simulink model "SquatTrotClimbRefined"  (R2025b)
settings: Solver=ode45  StartTime=0.0  StopTime=200  MaxStep=0.002  RelTol=0.01  AbsTol=0.01  EnableMultiTasking=on
undefined symbols (not defined in the file): a, b, c, waypoints, X, Y, Z
libraries: sm_lib x81, nesl_utility x67, hdlsllib x12, slpidlib x2, robotalgslib x1, sharedtransform x1
(part 4 of 6)

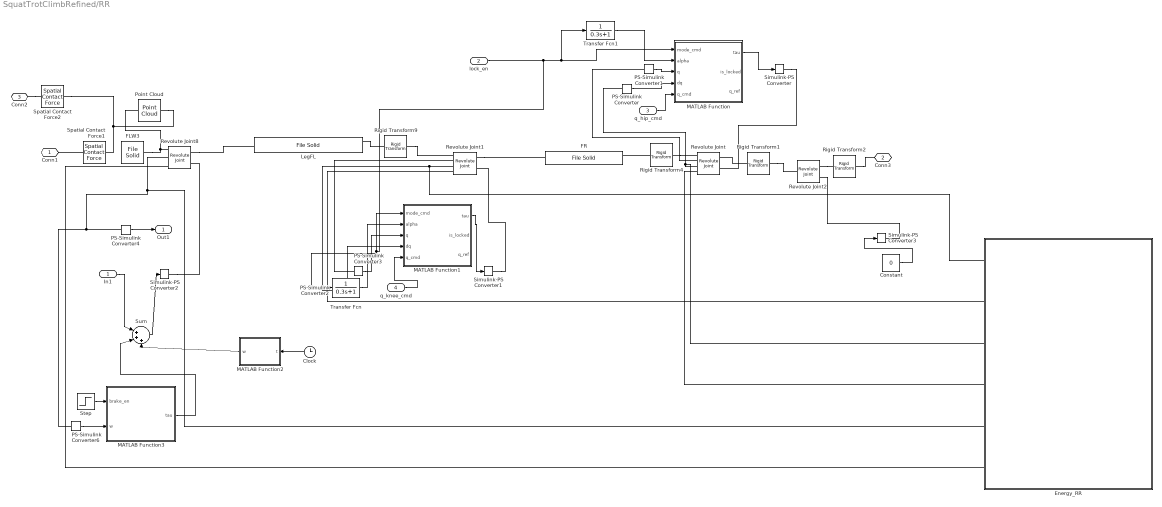
== system SquatTrotClimbRefined/RR ==
  In1 : Inport
  lock_en : Inport  Port=2
  q_hip_cmd : Inport  Port=3
  q_knee_cmd : Inport  Port=4
  Clock : Clock
  Constant : Constant  Value=0
  Energy_RR : Subsystem
  FLW3 : sm_lib/Body Elements/File Solid  ExtGeomFileName=Cheng Shin C-166-1.stp  UnitType=FromFile  ExtGeomFileUnits=m  StepReaderType=HEX  ExportConvexHullGeometry=on  InertiaType=CalculateFromGeometry  BasedOnType=Density  Density=400  DensityUnits=kg/m^3  Mass=1  MassUnits=kg  CenterOfMass=[0 0 0]  CenterOfMassUnits=m  MomentsOfInertia=[1 1 1]  MomentsOfInertiaUnits=kg*m^2  ProductsOfInertia=[0 0 0]  ProductsOfInertiaUnits=kg*m^2  GraphicType=FromGeometry  MarkerShape=Sphere  MarkerSize=10  GraphicVisPropType=AdvancedVisualProperties  GraphicDiffuseColor=[0.1 0.1 0.1]  GraphicOpacity=1  GraphicSpecularColor=[0.2 0.2 0.2 1.0]  GraphicAmbientColor=[0.05 0.05 0.05 1.0]  GraphicEmissiveColor=[0.0 0.0 0.0 1.0]  GraphicShininess=10  DoExposeReferenceFrame=off  SerializedFrames=<Frames><Frame><Id>Frame1</Id><Value><Name>F1</Name><Origin><Source>CenterOfMassFrame</Source><FeatureName>toroidal surface 99</FeatureName></Origin><PrimaryAxis><DefinedDirection>+Z</DefinedDirection><Source>ReferenceFrame</Source><SourceDirection>+Z</SourceDirection><FeatureName></FeatureName></PrimaryAxis><SecondaryAxis><DefinedDirection>+X</DefinedDirection><Source>ReferenceFrame</Source><SourceDirection>+X</SourceDirection><FeatureName></FeatureName></SecondaryAxis></Value></Frame></Frames>
  FR : sm_lib/Body Elements/File Solid  ExtGeomFileName=haut patte D.STEP  UnitType=FromFile  ExtGeomFileUnits=m  StepReaderType=HEX  ExportConvexHullGeometry=on  InertiaType=CalculateFromGeometry  BasedOnType=Density  Density=800  DensityUnits=kg/m^3  Mass=1  MassUnits=kg  CenterOfMass=[0 0 0]  CenterOfMassUnits=m  MomentsOfInertia=[1 1 1]  MomentsOfInertiaUnits=kg*m^2  ProductsOfInertia=[0 0 0]  ProductsOfInertiaUnits=kg*m^2  GraphicType=FromGeometry  MarkerShape=Sphere  MarkerSize=10  GraphicVisPropType=AdvancedVisualProperties  GraphicDiffuseColor=[0.9 0.9 0.9]  GraphicOpacity=1  GraphicSpecularColor=[0.9 0.9 0.9 1.0]  GraphicAmbientColor=[0.1 0.1 0.1 1.0]  GraphicEmissiveColor=[0.0 0.0 0.0 1.0]  GraphicShininess=100  DoExposeReferenceFrame=off  SerializedFrames=<Frames><Frame><Id>Frame1</Id><Value><Name>H-L link</Name><Origin><Source>GeometricFeature</Source><FeatureName>spherical surface 2</FeatureName></Origin><PrimaryAxis><DefinedDirection>+Z</DefinedDirection><Source>ReferenceFrame</Source><SourceDirection>+Z</SourceDirection><FeatureName></FeatureName></PrimaryAxis><SecondaryAxis><DefinedDirection>+X</DefinedDirection><Source>ReferenceFrame</Source><SourceDirection>-Y</SourceDirection><FeatureName></FeatureName></SecondaryAxis></Value></Frame><Frame><Id>Frame2</Id><Value><Name>L-K link</Name><Origin><Source>GeometricFeature</Source><FeatureName>cylindrical surface 2</FeatureName></Origin><PrimaryAxis><DefinedDirection>+Z</DefinedDirection><Source>ReferenceFrame</Source><SourceDirection>+Z</SourceDirection><FeatureName></FeatureName></PrimaryAxis><SecondaryAxis><DefinedDirection>+X</DefinedDirection><Source>ReferenceFrame</Source><SourceDirection>-Y</SourceDirection><FeatureName></FeatureName></SecondaryAxis></Value></Frame></Frames>
  LegFL : sm_lib/Body Elements/File Solid  ExtGeomFileName=leg.STEP  UnitType=FromFile  ExtGeomFileUnits=m  StepReaderType=HEX  ExportConvexHullGeometry=on  InertiaType=CalculateFromGeometry  BasedOnType=Density  Density=800  DensityUnits=kg/m^3  Mass=1  MassUnits=kg  CenterOfMass=[0 0 0]  CenterOfMassUnits=m  MomentsOfInertia=[1 1 1]  MomentsOfInertiaUnits=kg*m^2  ProductsOfInertia=[0 0 0]  ProductsOfInertiaUnits=kg*m^2  GraphicType=FromGeometry  MarkerShape=Sphere  MarkerSize=10  GraphicVisPropType=AdvancedVisualProperties  GraphicDiffuseColor=[0 0 0]  GraphicOpacity=1  GraphicSpecularColor=[0.9 0.9 0.9 1.0]  GraphicAmbientColor=[0.1 0.1 0.1 1.0]  GraphicEmissiveColor=[0.0 0.0 0.0 1.0]  GraphicShininess=100  DoExposeReferenceFrame=off  SerializedFrames=|
      | <Frames>
      | 
      |   <Frame>
      |     <Id>Frame1</Id>
      |     <Value>
      |       <Name>L-K link</Name>
      |       <Origin>
      |         <Source>GeometricFeature</Source>
      |         <FeatureName>cylindrical surface 6</FeatureName>
      |       </Origin>
      |       <PrimaryAxis>
      |         <DefinedDirection>+Z</DefinedDirection>
      |         <Source>ReferenceFrame</Source>
      |         <SourceDirection>+Z</SourceDirection>
      |         <FeatureName></FeatureName>
      |       </PrimaryAxis>
      |       <SecondaryAxis>
      |         <DefinedDirection>+X</DefinedDirection>
      |         <Source>ReferenceFrame</Source>
      |         <SourceDirection>-X</SourceDirection>
      |         <FeatureName></FeatureName>
      |       </SecondaryAxis>
      |     </Value>
      |   </Frame>
      | 
      |   <Frame>
      |     <Id>Frame2</Id>
      |     <Value>
      |       <Name>L-W link</Name>
      |       <Origin>
      |         <Source>GeometricFeature</Source>
      |         <FeatureName>cylindrical surface 4</FeatureName>
      |       </Origin>
      |       <PrimaryAxis>
      |         <DefinedDirection>+Z</DefinedDirection>
      |         <Source>ReferenceFrame</Source>
      |         <SourceDirection>+Z</SourceDirection>
      |         <FeatureName></FeatureName>
      |       </PrimaryAxis>
      |       <SecondaryAxis>
      |         <DefinedDirection>+X</DefinedDirection>
      |         <Source>ReferenceFrame</Source>
      |         <SourceDirection>-X</SourceDirection>
      |         <FeatureName></FeatureName>
      |       </SecondaryAxis>
      |     </Value>
      |   </Frame>
      | 
      | </Frames>
  MATLAB Function : MATLAB Function  TreatAsAtomicUnit=on  SystemSampleTime=0.002
  MATLAB Function1 : MATLAB Function  TreatAsAtomicUnit=on  SystemSampleTime=0.002
  MATLAB Function2 : MATLAB Function  TreatAsAtomicUnit=on
  MATLAB Function3 : MATLAB Function  TreatAsAtomicUnit=on
  PS-Simulink Converter{,1..4,6} (6 alike) : nesl_utility/PS-Simulink Converter  PhysicalDomain=network_engine_domain  SubClassName=ps_output  LeftPortType=input  RightPortType=output  PseudoPeriodic=off  Frequencies=[]  VectorFormat=inherit  Unit=inherit  AffineConversion=off
  Point Cloud : sm_lib/Curves and Surfaces/Point Cloud  CoordinatesMatrix=wheel_pts  CoordinatesMatrixUnits=m  GraphicType=MarkerCloud  GraphicSphereRadius=1e-2  GraphicSphereRadiusUnits=m  GraphicVisPropType=SimpleVisualProperties  GraphicDiffuseColor=[0.5 0.5 0.5]  GraphicOpacity=1  GraphicSpecularColor=[0.5 0.5 0.5 1.0]  GraphicAmbientColor=[0.15 0.15 0.15 1.0]  GraphicEmissiveColor=[0.0 0.0 0.0 1.0]  GraphicShininess=75
  Revolute Joint : sm_lib/Joints/Revolute Joint  JointMode=Normal  CompositeWrenchDir=FollowerOnBase  CompositeWrenchFrame=BaseFrame  SenseConstraintForce=off  SenseConstraintTorque=off  SenseTotalForce=off  SenseTotalTorque=off  PositionTargetSpecify=off  PositionTargetPriority=High  PositionTargetValue=0  PositionTargetValueUnits=deg  VelocityTargetSpecify=off  VelocityTargetPriority=High  VelocityTargetValue=0  VelocityTargetValueUnits=deg/s  EquilibriumPosition=0  EquilibriumPositionUnits=deg  SpringStiffness=0  SpringStiffnessUnits=N*m/deg  DampingCoefficient=0  DampingCoefficientUnits=N*m/(deg/s)  LowerLimitSpecify=off  LowerLimitBound=-90  LowerLimitBoundUnits=deg  LowerLimitStiffness=1e4  LowerLimitStiffnessUnits=N*m/deg  LowerLimitDamping=10  LowerLimitDampingUnits=N*m/(deg/s)  LowerLimitTransitionRegionWidth=0.1  LowerLimitTransitionRegionWidthUnits=deg  UpperLimitSpecify=off  UpperLimitBound=90  UpperLimitBoundUnits=deg  UpperLimitStiffness=1e4  UpperLimitStiffnessUnits=N*m/deg  UpperLimitDamping=10  UpperLimitDampingUnits=N*m/(deg/s)  UpperLimitTransitionRegionWidth=0.1  UpperLimitTransitionRegionWidthUnits=deg  TorqueActuationMode=InputTorque  MotionActuationMode=ComputedMotion  SensePosition=on  SenseVelocity=on  SenseAcceleration=off  SenseTorqueForce=on  SenseLowerLimitTorqueForce=off  SenseUpperLimitTorqueForce=off
  Revolute Joint1 : sm_lib/Joints/Revolute Joint  JointMode=Normal  CompositeWrenchDir=FollowerOnBase  CompositeWrenchFrame=BaseFrame  SenseConstraintForce=off  SenseConstraintTorque=off  SenseTotalForce=off  SenseTotalTorque=off  PositionTargetSpecify=off  PositionTargetPriority=High  PositionTargetValue=0  PositionTargetValueUnits=deg  VelocityTargetSpecify=off  VelocityTargetPriority=High  VelocityTargetValue=0  VelocityTargetValueUnits=deg/s  EquilibriumPosition=0  EquilibriumPositionUnits=deg  SpringStiffness=0  SpringStiffnessUnits=N*m/deg  DampingCoefficient=0  DampingCoefficientUnits=N*m/(deg/s)  LowerLimitSpecify=off  LowerLimitBound=-90  LowerLimitBoundUnits=deg  LowerLimitStiffness=1e4  LowerLimitStiffnessUnits=N*m/deg  LowerLimitDamping=10  LowerLimitDampingUnits=N*m/(deg/s)  LowerLimitTransitionRegionWidth=0.1  LowerLimitTransitionRegionWidthUnits=deg  UpperLimitSpecify=off  UpperLimitBound=90  UpperLimitBoundUnits=deg  UpperLimitStiffness=1e4  UpperLimitStiffnessUnits=N*m/deg  UpperLimitDamping=10  UpperLimitDampingUnits=N*m/(deg/s)  UpperLimitTransitionRegionWidth=0.1  UpperLimitTransitionRegionWidthUnits=deg  TorqueActuationMode=InputTorque  MotionActuationMode=ComputedMotion  SensePosition=on  SenseVelocity=on  SenseAcceleration=off  SenseTorqueForce=on  SenseLowerLimitTorqueForce=off  SenseUpperLimitTorqueForce=off
  Revolute Joint2 : sm_lib/Joints/Revolute Joint  JointMode=Normal  CompositeWrenchDir=FollowerOnBase  CompositeWrenchFrame=BaseFrame  SenseConstraintForce=off  SenseConstraintTorque=off  SenseTotalForce=off  SenseTotalTorque=off  PositionTargetSpecify=off  PositionTargetPriority=High  PositionTargetValue=0  PositionTargetValueUnits=deg  VelocityTargetSpecify=off  VelocityTargetPriority=High  VelocityTargetValue=0  VelocityTargetValueUnits=deg/s  EquilibriumPosition=0  EquilibriumPositionUnits=deg  SpringStiffness=0  SpringStiffnessUnits=N*m/deg  DampingCoefficient=0  DampingCoefficientUnits=N*m/(deg/s)  LowerLimitSpecify=off  LowerLimitBound=-90  LowerLimitBoundUnits=deg  LowerLimitStiffness=1e4  LowerLimitStiffnessUnits=N*m/deg  LowerLimitDamping=10  LowerLimitDampingUnits=N*m/(deg/s)  LowerLimitTransitionRegionWidth=0.1  LowerLimitTransitionRegionWidthUnits=deg  UpperLimitSpecify=off  UpperLimitBound=90  UpperLimitBoundUnits=deg  UpperLimitStiffness=1e4  UpperLimitStiffnessUnits=N*m/deg  UpperLimitDamping=10  UpperLimitDampingUnits=N*m/(deg/s)  UpperLimitTransitionRegionWidth=0.1  UpperLimitTransitionRegionWidthUnits=deg  TorqueActuationMode=ComputedTorque  MotionActuationMode=InputMotion  SensePosition=off  SenseVelocity=off  SenseAcceleration=off  SenseTorqueForce=off  SenseLowerLimitTorqueForce=off  SenseUpperLimitTorqueForce=off
  Revolute Joint8 : sm_lib/Joints/Revolute Joint  JointMode=Normal  CompositeWrenchDir=FollowerOnBase  CompositeWrenchFrame=BaseFrame  SenseConstraintForce=off  SenseConstraintTorque=off  SenseTotalForce=off  SenseTotalTorque=off  PositionTargetSpecify=off  PositionTargetPriority=High  PositionTargetValue=0  PositionTargetValueUnits=deg  VelocityTargetSpecify=off  VelocityTargetPriority=High  VelocityTargetValue=0  VelocityTargetValueUnits=deg/s  EquilibriumPosition=0  EquilibriumPositionUnits=deg  SpringStiffness=0  SpringStiffnessUnits=N*m/deg  DampingCoefficient=0  DampingCoefficientUnits=N*m/(deg/s)  LowerLimitSpecify=off  LowerLimitBound=-90  LowerLimitBoundUnits=deg  LowerLimitStiffness=1e4  LowerLimitStiffnessUnits=N*m/deg  LowerLimitDamping=10  LowerLimitDampingUnits=N*m/(deg/s)  LowerLimitTransitionRegionWidth=0.1  LowerLimitTransitionRegionWidthUnits=deg  UpperLimitSpecify=off  UpperLimitBound=90  UpperLimitBoundUnits=deg  UpperLimitStiffness=1e4  UpperLimitStiffnessUnits=N*m/deg  UpperLimitDamping=10  UpperLimitDampingUnits=N*m/(deg/s)  UpperLimitTransitionRegionWidth=0.1  UpperLimitTransitionRegionWidthUnits=deg  TorqueActuationMode=InputTorque  MotionActuationMode=ComputedMotion  SensePosition=off  SenseVelocity=on  SenseAcceleration=off  SenseTorqueForce=on  SenseLowerLimitTorqueForce=off  SenseUpperLimitTorqueForce=off
  Rigid Transform1 : sm_lib/Frames and Transforms/Rigid Transform  RotationMethod=AlignedAxes  FollAlignAxisA=+Z  BaseAlignAxisA=+Y  FollAlignAxisB=+X  BaseAlignAxisB=+X  RotationStandardAxis=+Z  RotationAngle=0  RotationAngleUnits=deg  RotationArbitraryAxis=[0 0 1]  RotationSequenceAxes=FollowerAxes  RotationSequence=XYX  RotationSequenceAngles=[0 0 0]  RotationSequenceAnglesUnits=deg  RotationMatrix=[1 0 0;0 1 0;0 0 1]  Quaternion=[1 0 0 0]  TranslationMethod=None  TranslationCartesianOffset=[0 0 0]  TranslationCartesianOffsetUnits=m  TranslationStandardAxis=+Z  TranslationStandardOffset=0  TranslationStandardOffsetUnits=m  TranslationROffset=0  TranslationROffsetUnits=m  TranslationThetaOffset=0  TranslationThetaOffsetUnits=deg  TranslationZOffset=0  TranslationZOffsetUnits=m
  Rigid Transform2 : sm_lib/Frames and Transforms/Rigid Transform  RotationMethod=AlignedAxes  FollAlignAxisA=+Y  BaseAlignAxisA=+Y  FollAlignAxisB=+Z  BaseAlignAxisB=+X  RotationStandardAxis=+Z  RotationAngle=0  RotationAngleUnits=deg  RotationArbitraryAxis=[0 0 1]  RotationSequenceAxes=FollowerAxes  RotationSequence=XYX  RotationSequenceAngles=[0 0 0]  RotationSequenceAnglesUnits=deg  RotationMatrix=[1 0 0;0 1 0;0 0 1]  Quaternion=[1 0 0 0]  TranslationMethod=None  TranslationCartesianOffset=[0 0 0]  TranslationCartesianOffsetUnits=m  TranslationStandardAxis=+Z  TranslationStandardOffset=0  TranslationStandardOffsetUnits=m  TranslationROffset=0  TranslationROffsetUnits=m  TranslationThetaOffset=0  TranslationThetaOffsetUnits=deg  TranslationZOffset=0  TranslationZOffsetUnits=m
  Rigid Transform4 : sm_lib/Frames and Transforms/Rigid Transform  RotationMethod=RotationSequence  FollAlignAxisA=+X  BaseAlignAxisA=+Y  FollAlignAxisB=+Y  BaseAlignAxisB=+Z  RotationStandardAxis=+Z  RotationAngle=0  RotationAngleUnits=deg  RotationArbitraryAxis=[0 0 1]  RotationSequenceAxes=FollowerAxes  RotationSequence=XYZ  RotationSequenceAngles=[0 0 -60]  RotationSequenceAnglesUnits=deg  RotationMatrix=[1 0 0;0 1 0;0 0 1]  Quaternion=[1 0 0 0]  TranslationMethod=None  TranslationCartesianOffset=[0 0 0]  TranslationCartesianOffsetUnits=m  TranslationStandardAxis=+Z  TranslationStandardOffset=0  TranslationStandardOffsetUnits=m  TranslationROffset=0  TranslationROffsetUnits=m  TranslationThetaOffset=0  TranslationThetaOffsetUnits=deg  TranslationZOffset=0  TranslationZOffsetUnits=m
  Rigid Transform9 : sm_lib/Frames and Transforms/Rigid Transform  RotationMethod=RotationSequence  FollAlignAxisA=+X  BaseAlignAxisA=+Y  FollAlignAxisB=+Y  BaseAlignAxisB=+Z  RotationStandardAxis=+Z  RotationAngle=0  RotationAngleUnits=deg  RotationArbitraryAxis=[0 0 1]  RotationSequenceAxes=FollowerAxes  RotationSequence=XYZ  RotationSequenceAngles=[0 0 -30]  RotationSequenceAnglesUnits=deg  RotationMatrix=[1 0 0;0 1 0;0 0 1]  Quaternion=[1 0 0 0]  TranslationMethod=None  TranslationCartesianOffset=[0 0 0]  TranslationCartesianOffsetUnits=m  TranslationStandardAxis=+Z  TranslationStandardOffset=0  TranslationStandardOffsetUnits=m  TranslationROffset=0  TranslationROffsetUnits=m  TranslationThetaOffset=0  TranslationThetaOffsetUnits=deg  TranslationZOffset=0  TranslationZOffsetUnits=m
  Simulink-PS Converter{,1..3} (4 alike) : nesl_utility/Simulink-PS Converter  PhysicalDomain=network_engine_domain  SubClassName=ps_input  LeftPortType=input  RightPortType=output  PseudoPeriodic=off  Frequencies=[]  NoiseDistribution=none  NoiseParameters=[]  Unit=1  AffineConversion=off  FilteringAndDerivatives=provide  SimscapeFilterOrder=1  InputFilterTimeConstant=0.001  UdotUserProvided=0
  Spatial Contact Force1 : sm_lib/Forces and Torques/Spatial Contact Force  SenseSeparationDistance=off  NormalForceType=SmoothSpringDamper  NormalStiffness=1e6  NormalStiffnessUnits=N/m  NormalDamping=1e3  NormalDampingUnits=N/(m/s)  NormalTransitionRegionWidth=1e-4  NormalTransitionRegionWidthUnits=m  FrictionType=SmoothStickSlip  CoefficientOfStaticFriction=0.9  CoefficientOfDynamicFriction=0.7  FrictionalCriticalVelocity=1e-3  FrictionalCriticalVelocityUnits=m/s  SenseContactSignal=off  SensePenetrationDepth=off  SenseNormalVelocity=off  SenseTangentialVelocity=off  SensingForceTorqueDirection=BaseOnFollower  SensingForceTorqueResolutionFrame=ContactFrame  SenseNormalForce=off  SenseNormalForceMagnitude=off  SenseNormalTorque=off  SenseFrictionalForce=off  SenseFrictionalForceMagnitude=off  SenseFrictionalTorque=off  SenseTotalForce=off  SenseTotalTorque=off  SenseContactBaseRotation=off  SenseContactBaseTranslation=off  SenseContactFollowerRotation=off  SenseContactFollowerTranslation=off  ZeroCrossDetectContactStartAndEnd=off
  Spatial Contact Force2 : sm_lib/Forces and Torques/Spatial Contact Force  SenseSeparationDistance=off  NormalForceType=SmoothSpringDamper  NormalStiffness=1e6  NormalStiffnessUnits=N/m  NormalDamping=1e3  NormalDampingUnits=N/(m/s)  NormalTransitionRegionWidth=1e-4  NormalTransitionRegionWidthUnits=m  FrictionType=SmoothStickSlip  CoefficientOfStaticFriction=0.9  CoefficientOfDynamicFriction=0.7  FrictionalCriticalVelocity=1e-3  FrictionalCriticalVelocityUnits=m/s  SenseContactSignal=off  SensePenetrationDepth=off  SenseNormalVelocity=off  SenseTangentialVelocity=off  SensingForceTorqueDirection=BaseOnFollower  SensingForceTorqueResolutionFrame=ContactFrame  SenseNormalForce=off  SenseNormalForceMagnitude=off  SenseNormalTorque=off  SenseFrictionalForce=off  SenseFrictionalForceMagnitude=off  SenseFrictionalTorque=off  SenseTotalForce=off  SenseTotalTorque=off  SenseContactBaseRotation=off  SenseContactBaseTranslation=off  SenseContactFollowerRotation=off  SenseContactFollowerTranslation=off  ZeroCrossDetectContactStartAndEnd=off
  Step : Step  Time=100  SampleTime=0
  Sum : Sum  Inputs=|+++
  Transfer Fcn : TransferFcn  Denominator=[0.3 1]
  Transfer Fcn1 : TransferFcn  Denominator=[0.3 1]
  Conn1 : PMIOPort  Side=Left
  Conn3 : PMIOPort  Port=2  Side=Right
  Conn2 : PMIOPort  Port=3  Side=Left
  Out1 : Outport
  wires:
  MATLAB Function/1(tau) -> Simulink-PS Converter/1
  PS-Simulink Converter3/1 -> MATLAB Function1/3(q)
  PS-Simulink Converter2/1 -> MATLAB Function1/4(dq)
  PS-Simulink Converter/1 -> MATLAB Function/4(dq)
  PS-Simulink Converter1/1 -> MATLAB Function/3(q)
  MATLAB Function1/1(tau) -> Simulink-PS Converter1/1
  PS-Simulink Converter4/1 -> Out1/1
  Transfer Fcn1/1 -> MATLAB Function/2(alpha)
  q_knee_cmd/1 -> MATLAB Function1/5(q_cmd)
  q_hip_cmd/1 -> MATLAB Function/5(q_cmd)
  PS-Simulink Converter6/1 -> MATLAB Function3/2(w)
  In1/1 -> Sum/1
  MATLAB Function3/1(tau) -> Sum/2
  Sum/1 -> Simulink-PS Converter2/1
  Transfer Fcn/1 -> MATLAB Function1/2(alpha)
  Step/1 -> MATLAB Function3/1(brake_en)
  Clock/1 -> MATLAB Function2/1(t)
  MATLAB Function2/1(w) -> Sum/3
  lock_en/1 -> Transfer Fcn/1, MATLAB Function1/1(mode_cmd), Transfer Fcn1/1, MATLAB Function/1(mode_cmd)
  Constant/1 -> Simulink-PS Converter3/1
  connections:
  Rigid Transform1/RConn1 -- Revolute Joint/LConn1
  Simulink-PS Converter1/RConn1 -- Revolute Joint1/LConn2
  Revolute Joint8/LConn1 -- LegFL/RConn1
  Rigid Transform4/LConn1 -- Revolute Joint/RConn1
  PS-Simulink Converter2/LConn1 -- Energy_RR/LConn1 -- Revolute Joint1/RConn3
  PS-Simulink Converter/LConn1 -- Energy_RR/LConn3 -- Revolute Joint/RConn3
  Revolute Joint1/RConn2 -- PS-Simulink Converter3/LConn1
  Simulink-PS Converter/RConn1 -- Revolute Joint/LConn2
  PS-Simulink Converter1/LConn1 -- Revolute Joint/RConn2
  Simulink-PS Converter2/RConn1 -- Revolute Joint8/LConn2
  PS-Simulink Converter4/LConn1 -- Energy_RR/LConn5 -- Revolute Joint8/RConn2 -- PS-Simulink Converter6/LConn1
  Spatial Contact Force1/LConn1 -- Conn1/RConn1
  FLW3/LConn1 -- Point Cloud/LConn1 -- Revolute Joint8/RConn1
  Point Cloud/RConn1 -- Spatial Contact Force1/RConn1 -- Spatial Contact Force2/RConn1
  Rigid Transform4/RConn1 -- FR/LConn1
  Revolute Joint1/LConn1 -- FR/RConn1
  Rigid Transform9/LConn1 -- Revolute Joint1/RConn1
  LegFL/LConn1 -- Rigid Transform9/RConn1
  Rigid Transform1/LConn1 -- Revolute Joint2/RConn1
  Revolute Joint2/LConn1 -- Rigid Transform2/RConn1
  Rigid Transform2/LConn1 -- Conn3/RConn1
  Revolute Joint2/LConn2 -- Simulink-PS Converter3/RConn1
  Conn2/RConn1 -- Spatial Contact Force2/LConn1
  Revolute Joint8/RConn3 -- Energy_RR/LConn6
  Revolute Joint/RConn4 -- Energy_RR/LConn4
  Revolute Joint1/RConn4 -- Energy_RR/LConn2

== system SquatTrotClimbRefined/Rear_left_gait ==
  mode_cmd : Inport
  t : Inport  Port=2
  Constant : Constant  Value=2
  MATLAB Function2 : MATLAB Function  TreatAsAtomicUnit=on
  MATLAB Function4 : MATLAB Function  TreatAsAtomicUnit=on
  q_hip_RR : Outport
  q_knee_RR : Outport  Port=2
  wires:
  t/1 -> MATLAB Function2/1(t), MATLAB Function4/1(t)
  mode_cmd/1 -> MATLAB Function2/3(mode_cmd), MATLAB Function4/3(mode_cmd)
  MATLAB Function2/1(q_hip) -> q_hip_RR/1
  MATLAB Function4/1(q_knee) -> q_knee_RR/1
  Constant/1 -> MATLAB Function2/2(leg_id), MATLAB Function4/2(leg_id)

== system SquatTrotClimbRefined/Rear_right_gait ==
  mode_cmd : Inport
  t : Inport  Port=2
  Constant : Constant  Value=3
  MATLAB Function2 : MATLAB Function  TreatAsAtomicUnit=on
  MATLAB Function3 : MATLAB Function  TreatAsAtomicUnit=on
  q_hip_RL : Outport
  q_knee_RL : Outport  Port=2
  wires:
  MATLAB Function2/1(q_hip) -> q_hip_RL/1
  mode_cmd/1 -> MATLAB Function2/3(mode_cmd), MATLAB Function3/3(mode_cmd)
  t/1 -> MATLAB Function2/1(t), MATLAB Function3/1(t)
  MATLAB Function3/1(q_knee) -> q_knee_RL/1
  Constant/1 -> MATLAB Function2/2(leg_id), MATLAB Function3/2(leg_id)

== system SquatTrotClimbRefined/Subsystem ==
  Mechanism Configuration : sm_lib/Utilities/Mechanism Configuration  UniformGravity=Constant  GravityVector=[0 0 -9.80665]  GravityVectorUnits=m/s^2  LinearizationDelta=0.001  JointModeTransitionNonlinearIterations=2
  Solver Configuration : nesl_utility/Solver Configuration  PhysicalDomain=network_engine_domain  SubClassName=solver  LeftPortType=input  RightPortType=generic  Tones=[]  Harmonics=[]  SimulateNoise=off  Profile=off  UseLocalSampling=off  EnableSwitchedLinearOptims=on  FrequencyDomain=off  UseCCode=off  RelTol=0.001  AbsTol=1e-06  MinStep=1e-09  ToWorkspace=off  RevertToSquareIcSolve=off  NumHomotopyIterations=100  PhasorMode=off  PhasorModeNumHarmonics=1  ConsistencySolver=NEWTON_XTOL_AFTER_FTOL  IndexReductionMethod=DerivativeReplacement  DoDC=off  ResidualTolerance=1e-09  ConsistencyTolSource=GLOBAL  ConsistencyAbsTol=0.001  ConsistencyRelTol=0.001  ConsistencyTolFactor=0.001  UseLocalSolver=off  LocalSolverChoice=NE_BACKWARD_EULER_ADVANCER  ResolveIndetEquations=on  FunctionEvalNumThread=1  LocalSolverSampleTime=0.001  DoFixedCost=off  MaxNonlinIter=3  MaxModeIter=2  ComputeImpulses=off  ImpulseIterations=2  LinearAlgebra=Sparse  LinearAlgebraNumThread=0  EquationFormulation=NE_TIME_EF  DelaysMemoryBudget=1024  AutomaticFiltering=on  FilteringTimeConstant=0.001  PartitionStorageMethod=AS_NEEDED  PartitionMemoryBudget=1024  PartitionMethod=FAST  MultibodyUseLocalSolver=off  MultibodyLocalSolverChoice=ODE1  MultibodyLocalSolverSampleTime=0.001
  World Frame : sm_lib/Frames and Transforms/World Frame
  port : PMIOPort  Side=Right
  connections:
  Solver Configuration/RConn1 -- port/RConn1 -- Mechanism Configuration/RConn1 -- World Frame/RConn1

== system SquatTrotClimbRefined/Subsystem5 ==
  In2 : Inport
  wR_cmd : Inport  Port=2
  PID Controller : slpidlib/PID Controller  Controller=PID  Form=Parallel  TimeDomain=Continuous-time  UseExternalTs=off  SampleTime=-1  IntegratorMethod=Forward Euler  FilterMethod=Forward Euler  ControllerParametersSource=internal  P=5  I=0  UseKiTs=off  D=0  UseExternalDerivativeSource=off  N=100  UseFilter=on  TunerSelectOption=Transfer Function Based (PID Tuner App)  InitialConditionSource=internal  InitialConditionForIntegrator=0  InitialConditionForFilter=0  DifferentiatorICPrevScaledInput=0  ExternalReset=none  TrackingMode=off  Kt=1  LimitOutput=off  SatLimitsSource=internal  UpperSaturationLimit=inf  LowerSaturationLimit=-inf  LinearizeAsGain=on  AntiWindupMode=none  Kb=1  LimitIntegrator=off  UpperIntegratorSaturationLimit=inf  LowerIntegratorSaturationLimit=-inf  POutMin=[]  POutMax=[]  IOutMin=[]  IOutMax=[]  DOutMin=[]  DOutMax=[]  NOutMin=[]  NOutMax=[]  SumOutMin=[]  SumOutMax=[]  SaturationOutMin=[]  SaturationOutMax=[]  PParamMin=[]  PParamMax=[]  IParamMin=[]  IParamMax=[]  DParamMin=[]  DParamMax=[]  NParamMin=[]  NParamMax=[]  KbParamMin=[]  KbParamMax=[]  KtParamMin=[]  KtParamMax=[]  KbOutMin=[]  KbOutMax=[]  KtOutMin=[]  KtOutMax=[]  IntegratorOutMin=[]  IntegratorOutMax=[]  FilterOutMin=[]  FilterOutMax=[]  SumI1OutMin=[]  SumI1OutMax=[]  SumI2OutMin=[]  SumI2OutMax=[]  SumI3OutMin=[]  SumI3OutMax=[]  SumI4OutMin=[]  SumI4OutMax=[]  SumDOutMin=[]  SumDOutMax=[]  DifferentiatorOutMin=[]  DifferentiatorOutMax=[]  FilterDiffOutCoefMin=[]  FilterDiffOutCoefMax=[]  ReciprocalOutMin=[]  ReciprocalOutMax=[]  SumDenOutMin=[]  SumDenOutMax=[]  SumNumOutMin=[]  SumNumOutMax=[]  DivideOutMin=[]  DivideOutMax=[]  UdiffTsProdOutMin=[]  UdiffTsProdOutMax=[]  NTsProdOutMin=[]  NTsProdOutMax=[]  UintegralTsProdOutMin=[]  UintegralTsProdOutMax=[]  UngainTsProdOutMin=[]  UngainTsProdOutMax=[]  ClampingZeroOutDataTypeStr=Inherit: Inherit via back propagation  ClampingZeroOutMin=[]  ClampingZeroOutMax=[]  FilterDenConstantOutDataTypeStr=Inherit: Inherit via back propagation  FilterDenConstantOutMin=[]  FilterDenConstantOutMax=[]  PCopyOutDataTypeStr=Inherit: Inherit via back propagation  PCopyOutMin=[]  PCopyOutMax=[]  NCopyOutDataTypeStr=Inherit: Inherit via back propagation  NCopyOutMin=[]  NCopyOutMax=[]  IntegratorContinuousStateAttributes=''  IntegratorStateMustResolveToSignalObject=off  IntegratorRTWStateStorageClass=Auto  FilterContinuousStateAttributes=''  FilterStateMustResolveToSignalObject=off  FilterRTWStateStorageClass=Auto  ParallelPVariant=InternalParameters  IdealPVariant=Disabled  IVariant=InternalParameters  DVariant=InternalParameters  IntegratorVariant=Continuous  SatVariant=Disabled  AWVariant=Passthrough  PCopyVariant=Disabled  TRVariant=Disabled  FdbkBlocksVariant=Forward  IdealPFdbkVariant=Disabled  SatFdbkVariant=Disabled  DerivativeFilterVariant=ContFilter  NVariant=InternalParameters  NCopyVariant=Disabled  FilterICVariant=InternalICsFilter  IntegratorICVariant=InternalICs  ExternalResetVariant=Disabled  TRSumVariant=Passthrough  SumFdbkVariant=Disabled  SumVariant=Sum_PID  TsampFilterVariant=InternalTs  TsampNgainVariant=Passthrough  TsampIntegralVariant=Disabled_SignalSpec  ExternalSaturationOutDataTypeStr=Inherit: Same as second input  DerivativeSourceVariant=ErrorSignal  PreIntVariant=InternalPreInt
  Saturation : Saturate  UpperLimit=5  LowerLimit=-5
  Subtract : Sum  Inputs=+-
  Out1 : Outport
  wires:
  In2/1 -> Subtract/2
  Subtract/1 -> PID Controller/1
  Saturation/1 -> Out1/1
  PID Controller/1 -> Saturation/1
  wR_cmd/1 -> Subtract/1

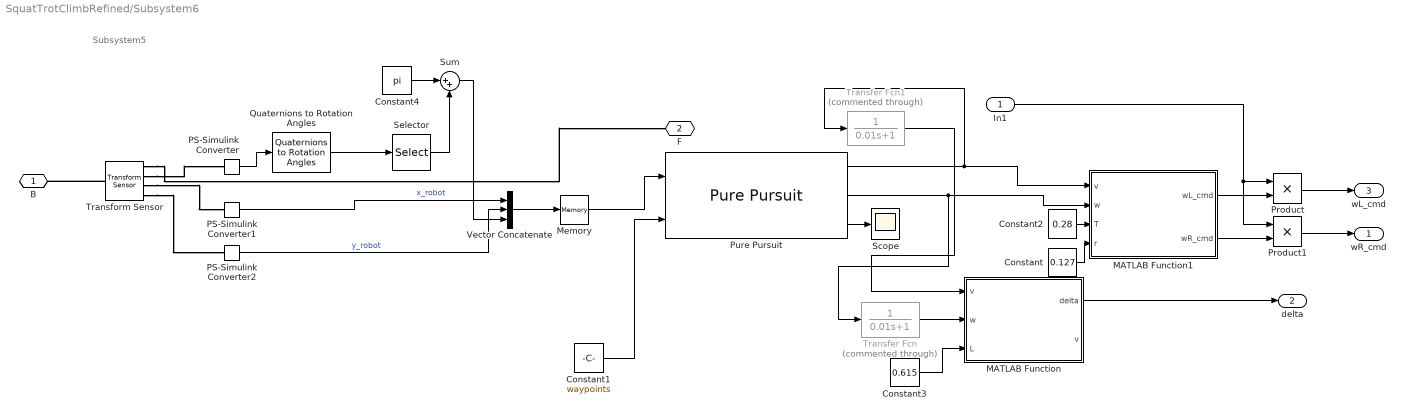
== system SquatTrotClimbRefined/Subsystem6 ==
  note: Subsystem5
  In1 : Inport
  Constant : Constant  Value=0.127
  Constant1 : Constant  Value=waypoints
  Constant2 : Constant  Value=0.28
  Constant3 : Constant  Value=0.615
  Constant4 : Constant  Value=pi
  MATLAB Function : MATLAB Function  TreatAsAtomicUnit=on
  MATLAB Function1 : MATLAB Function  TreatAsAtomicUnit=on
  Memory : Memory
  PS-Simulink Converter : nesl_utility/PS-Simulink Converter  PhysicalDomain=network_engine_domain  SubClassName=ps_output  LeftPortType=input  RightPortType=output  PseudoPeriodic=off  Frequencies=[]  VectorFormat=inherit  Unit=inherit  AffineConversion=off
  PS-Simulink Converter1 : nesl_utility/PS-Simulink Converter  PhysicalDomain=network_engine_domain  SubClassName=ps_output  LeftPortType=input  RightPortType=output  PseudoPeriodic=off  Frequencies=[]  VectorFormat=inherit  Unit=inherit  AffineConversion=off
  PS-Simulink Converter2 : nesl_utility/PS-Simulink Converter  PhysicalDomain=network_engine_domain  SubClassName=ps_output  LeftPortType=input  RightPortType=output  PseudoPeriodic=off  Frequencies=[]  VectorFormat=inherit  Unit=inherit  AffineConversion=off
  Product : Product
  Product1 : Product
  Pure Pursuit : robotalgslib/Pure Pursuit  DesiredLinearVelocityPort=off  DesiredLinearVelocity=0.7  MaxAngularVelocity=0.8  LookaheadDistancePort=off  LookaheadDistance=0.6  TargetDirPort=on  SimulateUsing=Code generation
      settings: LibrarySourceBlock=navlib/Control Algorithms/Pure Pursuit
  Quaternions to Rotation Angles : sharedtransform/Quaternions to Rotation Angles  rotationOrder=ZYX  aMode=aMode
  Scope : Scope
      settings: ActiveDisplayYMinimum=-49.938512022124293  ActiveDisplayYMaximum=229.50278461957694
  Selector : Selector  InputPortWidth=3  IndexOptions=Index vector (dialog)  Indices=[1]  OutputSizes=1
  Sum : Sum  Inputs=|++
  Transfer Fcn : TransferFcn  Commented=through  Denominator=[0.01 1]
  Transfer Fcn1 : TransferFcn  Commented=through  Denominator=[0.01 1]
  Transform Sensor : sm_lib/Frames and Transforms/Transform Sensor  MeasurementFrame=World  RotationSequence=XYX  SenseAngle=off  SenseAxis=off  SenseQ=on  SenseR=off  SenseRotationSequence=off  SenseOmegaX=off  SenseOmegaY=off  SenseOmegaZ=off  SenseOmega=off  SenseQDot=off  SenseRDot=off  SenseRotationSequenceDot=off  SenseAlphaX=off  SenseAlphaY=off  SenseAlphaZ=off  SenseAlpha=off  SenseQDDot=off  SenseRDDot=off  SenseX=on  SenseY=on  SenseZ=off  SenseXYZ=off  SenseRad=off  SenseAzim=off  SenseDist=off  SenseInc=off  SenseXDot=off  SenseYDot=off  SenseZDot=off  SenseXYZDot=off  SenseRadDot=off  SenseAzimDot=off  SenseDistDot=off  SenseIncDot=off  SenseXDDot=off  SenseYDDot=off  SenseZDDot=off  SenseXYZDDot=off  SenseRadDDot=off  SenseAzimDDot=off  SenseDistDDot=off  SenseIncDDot=off
  Vector Concatenate : Concatenate  NumInputs=3
  B : PMIOPort  Side=Right
  F : PMIOPort  Port=2  Side=Right
  wR_cmd : Outport
  delta : Outport  Port=2
  wL_cmd : Outport  Port=3
  wires:
  Pure Pursuit/2 -> MATLAB Function1/2(w), Transfer Fcn/1
  Transfer Fcn1/1 -> MATLAB Function/1("v ")
  Transfer Fcn/1 -> MATLAB Function/2(w)
  Constant1/1 -> Pure Pursuit/2
  Constant/1 -> MATLAB Function1/4(r)
  Constant2/1 -> MATLAB Function1/3(T)
  Constant3/1 -> MATLAB Function/3(L)
  Pure Pursuit/1 -> MATLAB Function1/1(v), Transfer Fcn1/1
  Pure Pursuit/3 -> Scope/1
  Memory/1 -> Pure Pursuit/1
  In1/1 -> Product/1, Product1/1
  MATLAB Function1/1(wL_cmd) -> Product/2
  Product/1 -> wL_cmd/1
  MATLAB Function1/2(wR_cmd) -> Product1/2
  Product1/1 -> wR_cmd/1
  MATLAB Function/1(delta) -> delta/1
  Sum/1 -> Vector Concatenate/3
  Selector/1 -> Sum/2
  Constant4/1 -> Sum/1
  PS-Simulink Converter2/1 -> Vector Concatenate/2  "y_robot"
  PS-Simulink Converter1/1 -> Vector Concatenate/1  "x_robot"
  Vector Concatenate/1 -> Memory/1
  PS-Simulink Converter/1 -> Quaternions to Rotation Angles/1
  Quaternions to Rotation Angles/1 -> Selector/1
  connections:
  Transform Sensor/RConn1 -- F/RConn1
  Transform Sensor/LConn1 -- B/RConn1
  Transform Sensor/RConn3 -- PS-Simulink Converter1/LConn1
  Transform Sensor/RConn2 -- PS-Simulink Converter/LConn1
  Transform Sensor/RConn4 -- PS-Simulink Converter2/LConn1

== system SquatTrotClimbRefined/Subsystem7 ==
  wL_cmd : Inport
  In2 : Inport  Port=2
  PID Controller : slpidlib/PID Controller  Controller=PID  Form=Parallel  TimeDomain=Continuous-time  UseExternalTs=off  SampleTime=-1  IntegratorMethod=Forward Euler  FilterMethod=Forward Euler  ControllerParametersSource=internal  P=5  I=0  UseKiTs=off  D=0  UseExternalDerivativeSource=off  N=100  UseFilter=on  TunerSelectOption=Transfer Function Based (PID Tuner App)  InitialConditionSource=internal  InitialConditionForIntegrator=0  InitialConditionForFilter=0  DifferentiatorICPrevScaledInput=0  ExternalReset=none  TrackingMode=off  Kt=1  LimitOutput=off  SatLimitsSource=internal  UpperSaturationLimit=inf  LowerSaturationLimit=-inf  LinearizeAsGain=on  AntiWindupMode=none  Kb=1  LimitIntegrator=off  UpperIntegratorSaturationLimit=inf  LowerIntegratorSaturationLimit=-inf  POutMin=[]  POutMax=[]  IOutMin=[]  IOutMax=[]  DOutMin=[]  DOutMax=[]  NOutMin=[]  NOutMax=[]  SumOutMin=[]  SumOutMax=[]  SaturationOutMin=[]  SaturationOutMax=[]  PParamMin=[]  PParamMax=[]  IParamMin=[]  IParamMax=[]  DParamMin=[]  DParamMax=[]  NParamMin=[]  NParamMax=[]  KbParamMin=[]  KbParamMax=[]  KtParamMin=[]  KtParamMax=[]  KbOutMin=[]  KbOutMax=[]  KtOutMin=[]  KtOutMax=[]  IntegratorOutMin=[]  IntegratorOutMax=[]  FilterOutMin=[]  FilterOutMax=[]  SumI1OutMin=[]  SumI1OutMax=[]  SumI2OutMin=[]  SumI2OutMax=[]  SumI3OutMin=[]  SumI3OutMax=[]  SumI4OutMin=[]  SumI4OutMax=[]  SumDOutMin=[]  SumDOutMax=[]  DifferentiatorOutMin=[]  DifferentiatorOutMax=[]  FilterDiffOutCoefMin=[]  FilterDiffOutCoefMax=[]  ReciprocalOutMin=[]  ReciprocalOutMax=[]  SumDenOutMin=[]  SumDenOutMax=[]  SumNumOutMin=[]  SumNumOutMax=[]  DivideOutMin=[]  DivideOutMax=[]  UdiffTsProdOutMin=[]  UdiffTsProdOutMax=[]  NTsProdOutMin=[]  NTsProdOutMax=[]  UintegralTsProdOutMin=[]  UintegralTsProdOutMax=[]  UngainTsProdOutMin=[]  UngainTsProdOutMax=[]  ClampingZeroOutDataTypeStr=Inherit: Inherit via back propagation  ClampingZeroOutMin=[]  ClampingZeroOutMax=[]  FilterDenConstantOutDataTypeStr=Inherit: Inherit via back propagation  FilterDenConstantOutMin=[]  FilterDenConstantOutMax=[]  PCopyOutDataTypeStr=Inherit: Inherit via back propagation  PCopyOutMin=[]  PCopyOutMax=[]  NCopyOutDataTypeStr=Inherit: Inherit via back propagation  NCopyOutMin=[]  NCopyOutMax=[]  IntegratorContinuousStateAttributes=''  IntegratorStateMustResolveToSignalObject=off  IntegratorRTWStateStorageClass=Auto  FilterContinuousStateAttributes=''  FilterStateMustResolveToSignalObject=off  FilterRTWStateStorageClass=Auto  ParallelPVariant=InternalParameters  IdealPVariant=Disabled  IVariant=InternalParameters  DVariant=InternalParameters  IntegratorVariant=Continuous  SatVariant=Disabled  AWVariant=Passthrough  PCopyVariant=Disabled  TRVariant=Disabled  FdbkBlocksVariant=Forward  IdealPFdbkVariant=Disabled  SatFdbkVariant=Disabled  DerivativeFilterVariant=ContFilter  NVariant=InternalParameters  NCopyVariant=Disabled  FilterICVariant=InternalICsFilter  IntegratorICVariant=InternalICs  ExternalResetVariant=Disabled  TRSumVariant=Passthrough  SumFdbkVariant=Disabled  SumVariant=Sum_PID  TsampFilterVariant=InternalTs  TsampNgainVariant=Passthrough  TsampIntegralVariant=Disabled_SignalSpec  ExternalSaturationOutDataTypeStr=Inherit: Same as second input  DerivativeSourceVariant=ErrorSignal  PreIntVariant=InternalPreInt
  Saturation : Saturate  UpperLimit=5  LowerLimit=-5
  Subtract : Sum  Inputs=+-
  Out1 : Outport
  wires:
  In2/1 -> Subtract/2
  Subtract/1 -> PID Controller/1
  Saturation/1 -> Out1/1
  PID Controller/1 -> Saturation/1
  wL_cmd/1 -> Subtract/1

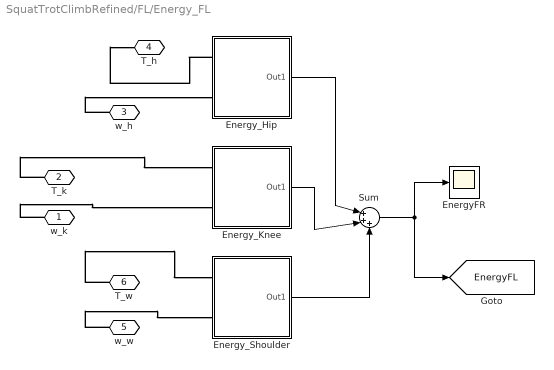
== system SquatTrotClimbRefined/FL/Energy_FL ==
  EnergyFR : Scope
  Energy_Hip : Subsystem
  Energy_Knee : Subsystem
  Energy_Shoulder : Subsystem
  Sum : Sum  Inputs=|+++
  w_k : PMIOPort  Side=Left
  T_k : PMIOPort  Port=2  Side=Left
  w_h : PMIOPort  Port=3  Side=Left
  T_h : PMIOPort  Port=4  Side=Left
  w_w : PMIOPort  Port=5  Side=Left
  T_w : PMIOPort  Port=6  Side=Left
  tag scope: EnergyFL=global
  wires:
  Energy_Knee/1(Out1) -> Sum/2
  Energy_Shoulder/1(Out1) -> Sum/3
  Energy_Hip/1(Out1) -> Sum/1
  Sum/1 -> EnergyFR/1, [EnergyFL]
  connections:
  T_w/RConn1 -- Energy_Shoulder/LConn1
  Energy_Hip/LConn1 -- T_h/RConn1
  w_k/RConn1 -- Energy_Knee/LConn2
  w_h/RConn1 -- Energy_Hip/LConn2
  w_w/RConn1 -- Energy_Shoulder/LConn2
  T_k/RConn1 -- Energy_Knee/LConn1

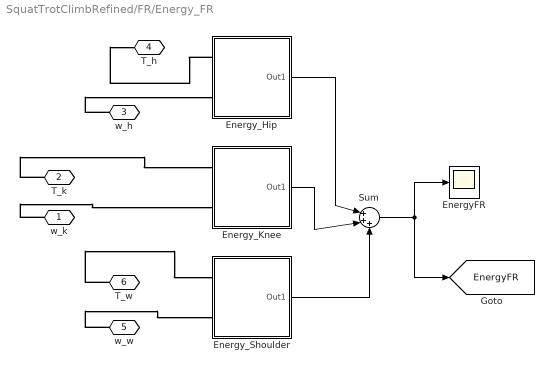
== system SquatTrotClimbRefined/FR/Energy_FR ==
  EnergyFR : Scope
  Energy_Hip : Subsystem
  Energy_Knee : Subsystem
  Energy_Shoulder : Subsystem
  Sum : Sum  Inputs=|+++
  w_k : PMIOPort  Side=Left
  T_k : PMIOPort  Port=2  Side=Left
  w_h : PMIOPort  Port=3  Side=Left
  T_h : PMIOPort  Port=4  Side=Left
  w_w : PMIOPort  Port=5  Side=Left
  T_w : PMIOPort  Port=6  Side=Left
  tag scope: EnergyFR=global
  wires:
  Energy_Knee/1(Out1) -> Sum/2
  Energy_Shoulder/1(Out1) -> Sum/3
  Energy_Hip/1(Out1) -> Sum/1
  Sum/1 -> EnergyFR/1, [EnergyFR]
  connections:
  T_w/RConn1 -- Energy_Shoulder/LConn1
  Energy_Hip/LConn1 -- T_h/RConn1
  w_k/RConn1 -- Energy_Knee/LConn2
  w_h/RConn1 -- Energy_Hip/LConn2
  w_w/RConn1 -- Energy_Shoulder/LConn2
  T_k/RConn1 -- Energy_Knee/LConn1

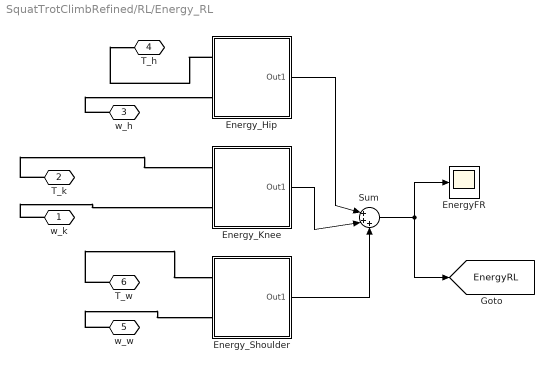
== system SquatTrotClimbRefined/RL/Energy_RL ==
  EnergyFR : Scope
  Energy_Hip : Subsystem
  Energy_Knee : Subsystem
  Energy_Shoulder : Subsystem
  Sum : Sum  Inputs=|+++
  w_k : PMIOPort  Side=Left
  T_k : PMIOPort  Port=2  Side=Left
  w_h : PMIOPort  Port=3  Side=Left
  T_h : PMIOPort  Port=4  Side=Left
  w_w : PMIOPort  Port=5  Side=Left
  T_w : PMIOPort  Port=6  Side=Left
  tag scope: EnergyRL=global
  wires:
  Energy_Knee/1(Out1) -> Sum/2
  Energy_Shoulder/1(Out1) -> Sum/3
  Energy_Hip/1(Out1) -> Sum/1
  Sum/1 -> EnergyFR/1, [EnergyRL]
  connections:
  T_w/RConn1 -- Energy_Shoulder/LConn1
  Energy_Hip/LConn1 -- T_h/RConn1
  w_k/RConn1 -- Energy_Knee/LConn2
  w_h/RConn1 -- Energy_Hip/LConn2
  w_w/RConn1 -- Energy_Shoulder/LConn2
  T_k/RConn1 -- Energy_Knee/LConn1

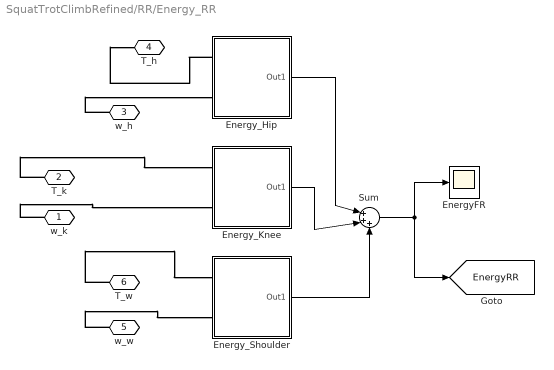
== system SquatTrotClimbRefined/RR/Energy_RR ==
  EnergyFR : Scope
      settings: ActiveDisplayYMinimum=-1  ActiveDisplayYMaximum=1
  Energy_Hip : Subsystem
  Energy_Knee : Subsystem
  Energy_Shoulder : Subsystem
  Sum : Sum  Inputs=|+++
  w_k : PMIOPort  Side=Left
  T_k : PMIOPort  Port=2  Side=Left
  w_h : PMIOPort  Port=3  Side=Left
  T_h : PMIOPort  Port=4  Side=Left
  w_w : PMIOPort  Port=5  Side=Left
  T_w : PMIOPort  Port=6  Side=Left
  tag scope: EnergyRR=global
  wires:
  Energy_Knee/1(Out1) -> Sum/2
  Energy_Shoulder/1(Out1) -> Sum/3
  Energy_Hip/1(Out1) -> Sum/1
  Sum/1 -> EnergyFR/1, [EnergyRR]
  connections:
  T_w/RConn1 -- Energy_Shoulder/LConn1
  Energy_Hip/LConn1 -- T_h/RConn1
  w_k/RConn1 -- Energy_Knee/LConn2
  w_h/RConn1 -- Energy_Hip/LConn2
  w_w/RConn1 -- Energy_Shoulder/LConn2
  T_k/RConn1 -- Energy_Knee/LConn1

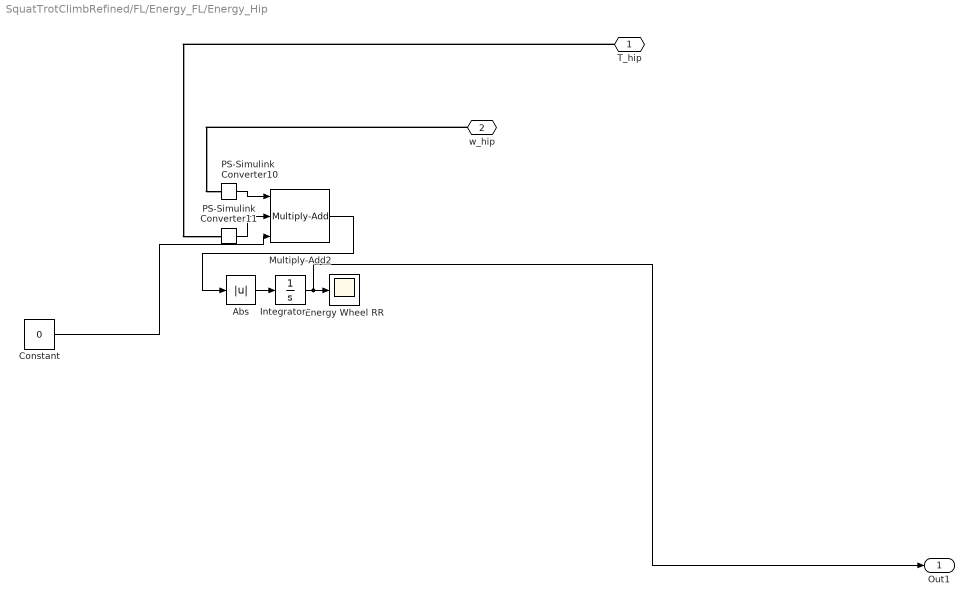
== system SquatTrotClimbRefined/FL/Energy_FL/Energy_Hip ==
  Abs : Abs  ZeroCross=off  SaturateOnIntegerOverflow=off
  Constant : Constant  Value=0
  Energy Wheel RR : Scope
      settings: ActiveDisplayYMinimum=-137.61876169666837  ActiveDisplayYMaximum=1238.5688552700155  DataLoggingVariableName=ScopeData3
  Integrator : Integrator
  Multiply-Add2 : hdlsllib/HDL Operations/Multiply-Add  Function=c+(a.*b)  datatype=Inherit: Inherit via internal rule  DoSatur=off  FMA=off
  PS-Simulink Converter10 : nesl_utility/PS-Simulink Converter  PhysicalDomain=network_engine_domain  SubClassName=ps_output  LeftPortType=input  RightPortType=output  PseudoPeriodic=off  Frequencies=[]  VectorFormat=inherit  Unit=inherit  AffineConversion=off
  PS-Simulink Converter11 : nesl_utility/PS-Simulink Converter  PhysicalDomain=network_engine_domain  SubClassName=ps_output  LeftPortType=input  RightPortType=output  PseudoPeriodic=off  Frequencies=[]  VectorFormat=inherit  Unit=inherit  AffineConversion=off
  T_hip : PMIOPort  Side=Left
  w_hip : PMIOPort  Port=2  Side=Left
  Out1 : Outport
  wires:
  Multiply-Add2/1 -> Abs/1
  Abs/1 -> Integrator/1
  Constant/1 -> Multiply-Add2/3
  PS-Simulink Converter11/1 -> Multiply-Add2/2
  Integrator/1 -> Energy Wheel RR/1, Out1/1
  PS-Simulink Converter10/1 -> Multiply-Add2/1
  connections:
  w_hip/RConn1 -- PS-Simulink Converter10/LConn1
  T_hip/RConn1 -- PS-Simulink Converter11/LConn1

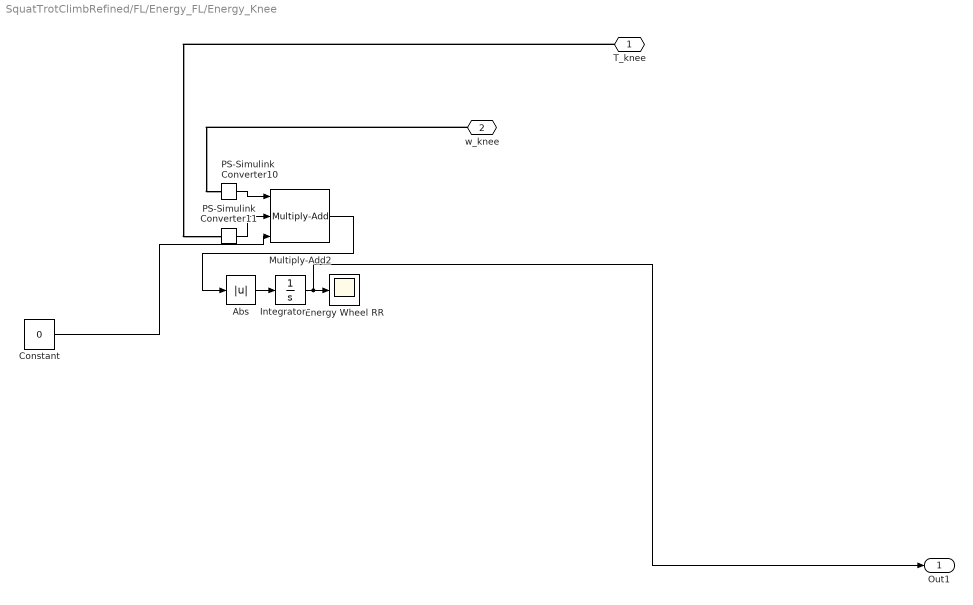
== system SquatTrotClimbRefined/FL/Energy_FL/Energy_Knee ==
  Abs : Abs  ZeroCross=off  SaturateOnIntegerOverflow=off
  Constant : Constant  Value=0
  Energy Wheel RR : Scope
      settings: ActiveDisplayYMinimum=-4.4698446843183612  ActiveDisplayYMaximum=40.228602158865257  DataLoggingVariableName=ScopeData3
  Integrator : Integrator
  Multiply-Add2 : hdlsllib/HDL Operations/Multiply-Add  Function=c+(a.*b)  datatype=Inherit: Inherit via internal rule  DoSatur=off  FMA=off
  PS-Simulink Converter10 : nesl_utility/PS-Simulink Converter  PhysicalDomain=network_engine_domain  SubClassName=ps_output  LeftPortType=input  RightPortType=output  PseudoPeriodic=off  Frequencies=[]  VectorFormat=inherit  Unit=inherit  AffineConversion=off
  PS-Simulink Converter11 : nesl_utility/PS-Simulink Converter  PhysicalDomain=network_engine_domain  SubClassName=ps_output  LeftPortType=input  RightPortType=output  PseudoPeriodic=off  Frequencies=[]  VectorFormat=inherit  Unit=inherit  AffineConversion=off
  T_knee : PMIOPort  Side=Left
  w_knee : PMIOPort  Port=2  Side=Left
  Out1 : Outport
  wires:
  PS-Simulink Converter10/1 -> Multiply-Add2/1
  Integrator/1 -> Out1/1, Energy Wheel RR/1
  PS-Simulink Converter11/1 -> Multiply-Add2/2
  Constant/1 -> Multiply-Add2/3
  Abs/1 -> Integrator/1
  Multiply-Add2/1 -> Abs/1
  connections:
  T_knee/RConn1 -- PS-Simulink Converter11/LConn1
  w_knee/RConn1 -- PS-Simulink Converter10/LConn1

== system SquatTrotClimbRefined/FL/Energy_FL/Energy_Shoulder ==
  Abs : Abs  ZeroCross=off  SaturateOnIntegerOverflow=off
  Constant : Constant  Value=0
  Energy Wheel RR : Scope
      settings: ActiveDisplayYMinimum=-137.61876169666837  ActiveDisplayYMaximum=1238.5688552700155  DataLoggingVariableName=ScopeData3
  Integrator : Integrator
  Multiply-Add2 : hdlsllib/HDL Operations/Multiply-Add  Function=c+(a.*b)  datatype=Inherit: Inherit via internal rule  DoSatur=off  FMA=off
  PS-Simulink Converter10 : nesl_utility/PS-Simulink Converter  PhysicalDomain=network_engine_domain  SubClassName=ps_output  LeftPortType=input  RightPortType=output  PseudoPeriodic=off  Frequencies=[]  VectorFormat=inherit  Unit=inherit  AffineConversion=off
  PS-Simulink Converter11 : nesl_utility/PS-Simulink Converter  PhysicalDomain=network_engine_domain  SubClassName=ps_output  LeftPortType=input  RightPortType=output  PseudoPeriodic=off  Frequencies=[]  VectorFormat=inherit  Unit=inherit  AffineConversion=off
  T_Wheel : PMIOPort  Side=Left
  w_wheel : PMIOPort  Port=2  Side=Left
  Out1 : Outport
  wires:
  Multiply-Add2/1 -> Abs/1
  Abs/1 -> Integrator/1
  Constant/1 -> Multiply-Add2/3
  PS-Simulink Converter11/1 -> Multiply-Add2/2
  Integrator/1 -> Energy Wheel RR/1, Out1/1
  PS-Simulink Converter10/1 -> Multiply-Add2/1
  connections:
  w_wheel/RConn1 -- PS-Simulink Converter10/LConn1
  T_Wheel/RConn1 -- PS-Simulink Converter11/LConn1

== system SquatTrotClimbRefined/FR/Energy_FR/Energy_Hip ==
  Abs : Abs  ZeroCross=off  SaturateOnIntegerOverflow=off
  Constant : Constant  Value=0
  Energy Wheel RR : Scope
      settings: ActiveDisplayYMinimum=-137.61876169666837  ActiveDisplayYMaximum=1238.5688552700155  DataLoggingVariableName=ScopeData3
  Integrator : Integrator
  Multiply-Add2 : hdlsllib/HDL Operations/Multiply-Add  Function=c+(a.*b)  datatype=Inherit: Inherit via internal rule  DoSatur=off  FMA=off
  PS-Simulink Converter10 : nesl_utility/PS-Simulink Converter  PhysicalDomain=network_engine_domain  SubClassName=ps_output  LeftPortType=input  RightPortType=output  PseudoPeriodic=off  Frequencies=[]  VectorFormat=inherit  Unit=inherit  AffineConversion=off
  PS-Simulink Converter11 : nesl_utility/PS-Simulink Converter  PhysicalDomain=network_engine_domain  SubClassName=ps_output  LeftPortType=input  RightPortType=output  PseudoPeriodic=off  Frequencies=[]  VectorFormat=inherit  Unit=inherit  AffineConversion=off
  T_hip : PMIOPort  Side=Left
  w_hip : PMIOPort  Port=2  Side=Left
  Out1 : Outport
  wires:
  Multiply-Add2/1 -> Abs/1
  Abs/1 -> Integrator/1
  Constant/1 -> Multiply-Add2/3
  PS-Simulink Converter11/1 -> Multiply-Add2/2
  Integrator/1 -> Energy Wheel RR/1, Out1/1
  PS-Simulink Converter10/1 -> Multiply-Add2/1
  connections:
  w_hip/RConn1 -- PS-Simulink Converter10/LConn1
  T_hip/RConn1 -- PS-Simulink Converter11/LConn1

== system SquatTrotClimbRefined/FR/Energy_FR/Energy_Knee ==
  Abs : Abs  ZeroCross=off  SaturateOnIntegerOverflow=off
  Constant : Constant  Value=0
  Energy Wheel RR : Scope
      settings: ActiveDisplayYMinimum=-137.61876169666837  ActiveDisplayYMaximum=1238.5688552700155  DataLoggingVariableName=ScopeData3
  Integrator : Integrator
  Multiply-Add2 : hdlsllib/HDL Operations/Multiply-Add  Function=c+(a.*b)  datatype=Inherit: Inherit via internal rule  DoSatur=off  FMA=off
  PS-Simulink Converter10 : nesl_utility/PS-Simulink Converter  PhysicalDomain=network_engine_domain  SubClassName=ps_output  LeftPortType=input  RightPortType=output  PseudoPeriodic=off  Frequencies=[]  VectorFormat=inherit  Unit=inherit  AffineConversion=off
  PS-Simulink Converter11 : nesl_utility/PS-Simulink Converter  PhysicalDomain=network_engine_domain  SubClassName=ps_output  LeftPortType=input  RightPortType=output  PseudoPeriodic=off  Frequencies=[]  VectorFormat=inherit  Unit=inherit  AffineConversion=off
  T_knee : PMIOPort  Side=Left
  w_knee : PMIOPort  Port=2  Side=Left
  Out1 : Outport
  wires:
  PS-Simulink Converter10/1 -> Multiply-Add2/1
  Integrator/1 -> Out1/1, Energy Wheel RR/1
  PS-Simulink Converter11/1 -> Multiply-Add2/2
  Constant/1 -> Multiply-Add2/3
  Abs/1 -> Integrator/1
  Multiply-Add2/1 -> Abs/1
  connections:
  T_knee/RConn1 -- PS-Simulink Converter11/LConn1
  w_knee/RConn1 -- PS-Simulink Converter10/LConn1

== system SquatTrotClimbRefined/FR/Energy_FR/Energy_Shoulder ==
  Abs : Abs  ZeroCross=off  SaturateOnIntegerOverflow=off
  Constant : Constant  Value=0
  Energy Wheel RR : Scope
      settings: ActiveDisplayYMinimum=-137.61876169666837  ActiveDisplayYMaximum=1238.5688552700155  DataLoggingVariableName=ScopeData3
  Integrator : Integrator
  Multiply-Add2 : hdlsllib/HDL Operations/Multiply-Add  Function=c+(a.*b)  datatype=Inherit: Inherit via internal rule  DoSatur=off  FMA=off
  PS-Simulink Converter10 : nesl_utility/PS-Simulink Converter  PhysicalDomain=network_engine_domain  SubClassName=ps_output  LeftPortType=input  RightPortType=output  PseudoPeriodic=off  Frequencies=[]  VectorFormat=inherit  Unit=inherit  AffineConversion=off
  PS-Simulink Converter11 : nesl_utility/PS-Simulink Converter  PhysicalDomain=network_engine_domain  SubClassName=ps_output  LeftPortType=input  RightPortType=output  PseudoPeriodic=off  Frequencies=[]  VectorFormat=inherit  Unit=inherit  AffineConversion=off
  T_Wheel : PMIOPort  Side=Left
  w_wheel : PMIOPort  Port=2  Side=Left
  Out1 : Outport
  wires:
  Multiply-Add2/1 -> Abs/1
  Abs/1 -> Integrator/1
  Constant/1 -> Multiply-Add2/3
  PS-Simulink Converter11/1 -> Multiply-Add2/2
  Integrator/1 -> Energy Wheel RR/1, Out1/1
  PS-Simulink Converter10/1 -> Multiply-Add2/1
  connections:
  w_wheel/RConn1 -- PS-Simulink Converter10/LConn1
  T_Wheel/RConn1 -- PS-Simulink Converter11/LConn1

== system SquatTrotClimbRefined/RL/Energy_RL/Energy_Hip ==
  Abs : Abs  ZeroCross=off  SaturateOnIntegerOverflow=off
  Constant : Constant  Value=0
  Energy Wheel RR : Scope
      settings: ActiveDisplayYMinimum=-137.61876169666837  ActiveDisplayYMaximum=1238.5688552700155  DataLoggingVariableName=ScopeData3
  Integrator : Integrator
  Multiply-Add2 : hdlsllib/HDL Operations/Multiply-Add  Function=c+(a.*b)  datatype=Inherit: Inherit via internal rule  DoSatur=off  FMA=off
  PS-Simulink Converter10 : nesl_utility/PS-Simulink Converter  PhysicalDomain=network_engine_domain  SubClassName=ps_output  LeftPortType=input  RightPortType=output  PseudoPeriodic=off  Frequencies=[]  VectorFormat=inherit  Unit=inherit  AffineConversion=off
  PS-Simulink Converter11 : nesl_utility/PS-Simulink Converter  PhysicalDomain=network_engine_domain  SubClassName=ps_output  LeftPortType=input  RightPortType=output  PseudoPeriodic=off  Frequencies=[]  VectorFormat=inherit  Unit=inherit  AffineConversion=off
  T_hip : PMIOPort  Side=Left
  w_hip : PMIOPort  Port=2  Side=Left
  Out1 : Outport
  wires:
  Multiply-Add2/1 -> Abs/1
  Abs/1 -> Integrator/1
  Constant/1 -> Multiply-Add2/3
  PS-Simulink Converter11/1 -> Multiply-Add2/2
  Integrator/1 -> Energy Wheel RR/1, Out1/1
  PS-Simulink Converter10/1 -> Multiply-Add2/1
  connections:
  w_hip/RConn1 -- PS-Simulink Converter10/LConn1
  T_hip/RConn1 -- PS-Simulink Converter11/LConn1

== system SquatTrotClimbRefined/RL/Energy_RL/Energy_Knee ==
  Abs : Abs  ZeroCross=off  SaturateOnIntegerOverflow=off
  Constant : Constant  Value=0
  Energy Wheel RR : Scope
      settings: ActiveDisplayYMinimum=-137.61876169666837  ActiveDisplayYMaximum=1238.5688552700155  DataLoggingVariableName=ScopeData3
  Integrator : Integrator
  Multiply-Add2 : hdlsllib/HDL Operations/Multiply-Add  Function=c+(a.*b)  datatype=Inherit: Inherit via internal rule  DoSatur=off  FMA=off
  PS-Simulink Converter10 : nesl_utility/PS-Simulink Converter  PhysicalDomain=network_engine_domain  SubClassName=ps_output  LeftPortType=input  RightPortType=output  PseudoPeriodic=off  Frequencies=[]  VectorFormat=inherit  Unit=inherit  AffineConversion=off
  PS-Simulink Converter11 : nesl_utility/PS-Simulink Converter  PhysicalDomain=network_engine_domain  SubClassName=ps_output  LeftPortType=input  RightPortType=output  PseudoPeriodic=off  Frequencies=[]  VectorFormat=inherit  Unit=inherit  AffineConversion=off
  T_knee : PMIOPort  Side=Left
  w_knee : PMIOPort  Port=2  Side=Left
  Out1 : Outport
  wires:
  PS-Simulink Converter10/1 -> Multiply-Add2/1
  Integrator/1 -> Out1/1, Energy Wheel RR/1
  PS-Simulink Converter11/1 -> Multiply-Add2/2
  Constant/1 -> Multiply-Add2/3
  Abs/1 -> Integrator/1
  Multiply-Add2/1 -> Abs/1
  connections:
  T_knee/RConn1 -- PS-Simulink Converter11/LConn1
  w_knee/RConn1 -- PS-Simulink Converter10/LConn1
